simulink model "rmspec"  (Simulink 7.0)
settings: Solver=ode45  StartTime=0.0  StopTime=200  RelTol=1e-3
undefined symbols (not defined in the file): pfb_coeff_gen_calc
libraries: xbsIndex_r4 x3092, casper_library x230, xps_library x24
(part 3 of 33)

== system rmspec/stg3_isel ==
  sync_tvg : Inport
  tvg0 : Inport  Port=2
  tvg1 : Inport  Port=3
  sync_p : Inport  Port=4
  p0 : Inport  Port=5
  p1 : Inport  Port=6
  Constant13 : xbsIndex_r4/Constant  arith_type=Unsigned  const=1  n_bits=32  bin_pt=0  explicit_period=on  period=1  equ=P=C  opselect=C  inp2=PCIN>>17  opr=+  inp1=P  carry=CIN  dbl_ovrd=off  block_type=constant
  Delay1 : xbsIndex_r4/Delay  en=off  latency=1  dbl_ovrd=off  reg_retiming=off  block_type=delay
  Delay24 : xbsIndex_r4/Delay  en=off  latency=1  dbl_ovrd=off  reg_retiming=off  block_type=delay
  Delay3 : xbsIndex_r4/Delay  en=off  latency=1  dbl_ovrd=off  reg_retiming=off  block_type=delay
  Mux : xbsIndex_r4/Mux  inputs=2  en=off  latency=0  precision=Full  arith_type=Unsigned  n_bits=16  bin_pt=14  quantization=Truncate  overflow=Wrap  dbl_ovrd=off  block_type=mux
  Mux1 : xbsIndex_r4/Mux  inputs=2  en=off  latency=0  precision=Full  arith_type=Unsigned  n_bits=16  bin_pt=14  quantization=Truncate  overflow=Wrap  dbl_ovrd=off  block_type=mux
  Mux2 : xbsIndex_r4/Mux  inputs=2  en=off  latency=0  precision=Full  arith_type=Unsigned  n_bits=16  bin_pt=14  quantization=Truncate  overflow=Wrap  dbl_ovrd=off  block_type=mux
  en : xps_library/software register  Tag=xps:sw_reg  SystemSampleTime=-1  io_dir=From Processor  arith_type=Unsigned  bitwidth=32  bin_pt=0  sample_period=1  gw_name=rmspec_stg3_isel_en_user_data_out
      link override pfb1_tv_tge0_rst_user_data_out: arith_type=Unsigned  n_bits=32  bin_pt=0  period=1
      link override pfb1_tv_tgeA_rst_reg_user_data_out: arith_type=Unsigned  n_bits=32  bin_pt=0  period=1
      link override pfb1_tv_tgeA_rst_user_data_out: arith_type=Unsigned  n_bits=32  bin_pt=0  period=1
      link override rmspec_stg3_isel_en_user_data_out: arith_type=Unsigned  n_bits=32  bin_pt=0  period=1
      link override roach_mspec_stg3_isel_en_user_data_out: arith_type=Unsigned  n_bits=32  bin_pt=0  period=1
      link override stg1_stg1_isel_tvg_en_user_data_out: arith_type=Unsigned  n_bits=32  bin_pt=0  period=1
  lsb : xbsIndex_r4/Slice  nbits=1  boolean_output=on  mode=Lower Bit Location + Width  bit1=0  base1=LSB of Input  bit0=0  base0=LSB of Input  dbl_ovrd=off  block_type=slice
      settings: infoedit="Extracts a given range of bits from each input sample and presents it at the output.  The output type is ordinarily unsigned with binary point at zero, but can be Boolean when the slice is one bit wide.<P><P>Hardware notes: In hardware this block costs nothing."  block_version=10.1.3
  sync_o : Outport
  o1 : Outport  Port=2
  o2 : Outport  Port=3
  wires:
  Delay24/1 -> sync_o/1
  [sel] -> Mux/1
  Mux/1 -> Delay24/1
  Delay1/1 -> o1/1
  [sel] -> Mux1/1
  Mux1/1 -> Delay1/1
  Delay3/1 -> o2/1
  [sel] -> Mux2/1
  Mux2/1 -> Delay3/1
  en/1 -> lsb/1
  Constant13/1 -> en/1
  lsb/1 -> [sel]
  p1/1 -> Mux2/2
  tvg1/1 -> Mux2/3
  p0/1 -> Mux1/2
  tvg0/1 -> Mux1/3
  sync_p/1 -> Mux/2
  sync_tvg/1 -> Mux/3

== system rmspec/sys ==
  Constant1 : xbsIndex_r4/Constant  arith_type=Unsigned  const=2^5-1  n_bits=5  bin_pt=0  explicit_period=on  period=1  equ=P=C  opselect=C  inp2=PCIN>>17  opr=+  inp1=P  carry=CIN  dbl_ovrd=off  block_type=constant
  Constant4 : Constant  Value=0  OutDataType=sfix(16)  OutScaling=2^0
  Constant5 : xbsIndex_r4/Constant  arith_type=Unsigned  const=2^5-2  n_bits=5  bin_pt=0  explicit_period=on  period=1  equ=P=C  opselect=C  inp2=PCIN>>17  opr=+  inp1=P  carry=CIN  dbl_ovrd=off  block_type=constant
  Delay18 : xbsIndex_r4/Delay  en=off  latency=1  dbl_ovrd=off  reg_retiming=off  block_type=delay
  Delay19 : xbsIndex_r4/Delay  en=off  latency=1  dbl_ovrd=off  reg_retiming=off  block_type=delay
  Relational : xbsIndex_r4/Relational  mode=a=b  en=off  latency=0  dbl_ovrd=off  block_type=relational
      settings: block_version=10.1.3
  Relational1 : xbsIndex_r4/Relational  mode=a!=b  en=off  latency=0  dbl_ovrd=off  block_type=relational
      settings: block_version=10.1.3
  Slice : xbsIndex_r4/Slice  nbits=1  boolean_output=on  mode=Lower Bit Location + Width  bit1=0  base1=MSB of Input  bit0=0  base0=LSB of Input  dbl_ovrd=off  block_type=slice
      settings: infoedit="Extracts a given range of bits from each input sample and presents it at the output.  The output type is ordinarily unsigned with binary point at zero, but can be Boolean when the slice is one bit wide.<P><P>Hardware notes: In hardware this block costs nothing."  block_version=10.1.3
  reset_reg : xps_library/software register  Tag=xps:sw_reg  SystemSampleTime=-1  io_dir=From Processor  arith_type=Unsigned  bitwidth=32  bin_pt=0  sample_period=1  gw_name=rmspec_sys_reset_reg_user_data_out
      link override qdr_vacc_dram_buf_tv_Subsystem_reset_reg_user_data_out: arith_type=Unsigned  n_bits=32  bin_pt=0  period=1
      link override qdr_vacc_dram_buf_tv_reset_reg_user_data_out: arith_type=Unsigned  n_bits=32  bin_pt=0  period=1
      link override qdr_vacc_dram_buf_tv_sys_reset_reg_user_data_out: arith_type=Unsigned  n_bits=32  bin_pt=0  period=1
      link override qdr_vacc_dram_buf_tv_tvg2_chan_user_data_out: arith_type=Unsigned  n_bits=32  bin_pt=0  period=1
      link override rmspec_sys_reset_reg_user_data_out: arith_type=Unsigned  n_bits=32  bin_pt=0  period=1
      link override roach_mspec_sys_reset_reg_user_data_out: arith_type=Unsigned  n_bits=32  bin_pt=0  period=1
      link override stg1_sys_reset_reg_user_data_out: arith_type=Unsigned  n_bits=32  bin_pt=0  period=1
      link override stg3_backup_sys_reset_reg_user_data_out: arith_type=Unsigned  n_bits=32  bin_pt=0  period=1
      link override stg3_sys_reset_reg_user_data_out: arith_type=Unsigned  n_bits=32  bin_pt=0  period=1
  sync_counter : xbsIndex_r4/Counter  cnt_type=Free Running  cnt_to=15  operation=Up  start_count=0  cnt_by_val=1  arith_type=Unsigned  n_bits=5  bin_pt=0  load_pin=off  rst=on  en=on  explicit_period=on  period=1  dbl_ovrd=off  use_behavioral_HDL=off  use_rpm=off  implementation=Fabric  block_type=counter
  sync : Outport
  rst : Outport  Port=2
  wires:
  sync_counter/1 -> Relational/1, Relational1/1
  Constant5/1 -> Relational/2
  Constant4/1 -> reset_reg/1
  reset_reg/1 -> Slice/1
  Relational/1 -> Delay19/1
  Slice/1 -> sync_counter/1, Delay18/1
  Constant1/1 -> Relational1/2
  Relational1/1 -> sync_counter/2
  Delay18/1 -> rst/1
  Delay19/1 -> sync/1

== system rmspec/tgeC_en ==
  vldi : Inport
  rst : Inport  Port=2
  last : Inport  Port=3
  Constant : xbsIndex_r4/Constant  arith_type=Boolean  const=1  n_bits=1  bin_pt=0  explicit_period=off  period=1  equ=P=C  opselect=C  inp2=PCIN>>17  opr=+  inp1=P  carry=CIN  dbl_ovrd=off  block_type=constant
  Logical : xbsIndex_r4/Logical  logical_function=AND  inputs=2  en=off  latency=0  precision=Full  arith_type=Unsigned  n_bits=16  bin_pt=0  align_bp=on  dbl_ovrd=off  block_type=logical
  Register : xbsIndex_r4/Register  init=0  rst=on  en=on  dbl_ovrd=off  block_type=register
  vldo : Outport
  wires:
  vldi/1 -> Logical/1
  Logical/1 -> vldo/1
  Constant/1 -> Register/1
  rst/1 -> Register/2
  last/1 -> Register/3
  Register/1 -> Logical/2

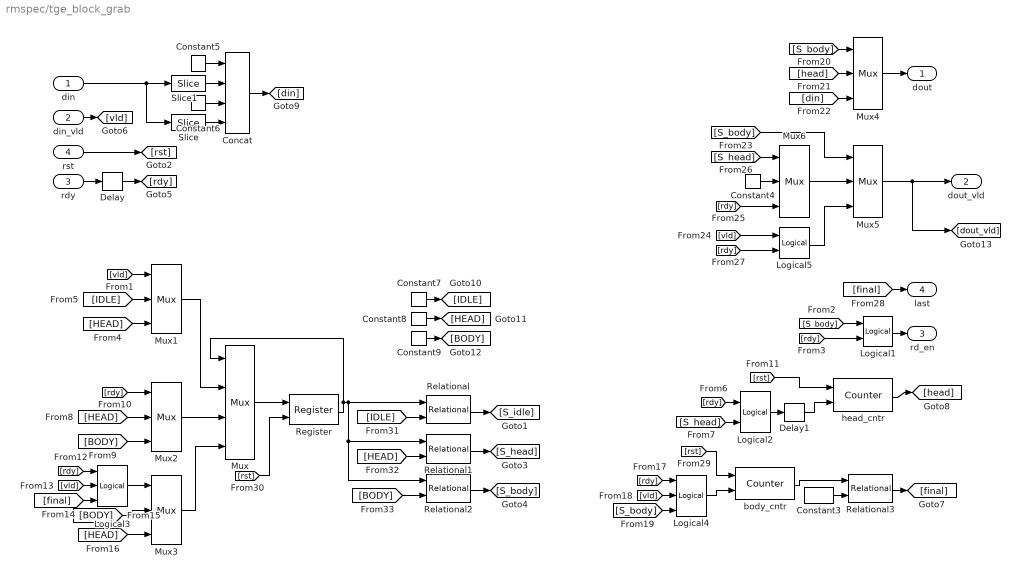
== system rmspec/tge_block_grab ==
  din : Inport
  din_vld : Inport  Port=2
  rdy : Inport  Port=3
  rst : Inport  Port=4
  Concat : xbsIndex_r4/Concat  num_inputs=4  dbl_ovrd=off  block_type=concat
      settings: block_version=10.1.3
  Constant3 : xbsIndex_r4/Constant  arith_type=Unsigned  const=2^9-1  n_bits=9  bin_pt=0  explicit_period=off  period=1  equ=P=C  opselect=C  inp2=PCIN>>17  opr=+  inp1=P  carry=CIN  dbl_ovrd=off  block_type=constant
  Constant4 : xbsIndex_r4/Constant  arith_type=Boolean  const=0  n_bits=2  bin_pt=0  explicit_period=off  period=1  equ=P=C  opselect=C  inp2=PCIN>>17  opr=+  inp1=P  carry=CIN  dbl_ovrd=off  block_type=constant
  Constant5 : xbsIndex_r4/Constant  arith_type=Unsigned  const=0  n_bits=14  bin_pt=0  explicit_period=off  period=1  equ=P=C  opselect=C  inp2=PCIN>>17  opr=+  inp1=P  carry=CIN  dbl_ovrd=off  block_type=constant
  Constant6 : xbsIndex_r4/Constant  arith_type=Unsigned  const=0  n_bits=14  bin_pt=0  explicit_period=off  period=1  equ=P=C  opselect=C  inp2=PCIN>>17  opr=+  inp1=P  carry=CIN  dbl_ovrd=off  block_type=constant
  Constant7 : xbsIndex_r4/Constant  arith_type=Unsigned  const=0  n_bits=2  bin_pt=0  explicit_period=off  period=1  equ=P=C  opselect=C  inp2=PCIN>>17  opr=+  inp1=P  carry=CIN  dbl_ovrd=off  block_type=constant
  Constant8 : xbsIndex_r4/Constant  arith_type=Unsigned  const=1  n_bits=2  bin_pt=0  explicit_period=off  period=1  equ=P=C  opselect=C  inp2=PCIN>>17  opr=+  inp1=P  carry=CIN  dbl_ovrd=off  block_type=constant
  Constant9 : xbsIndex_r4/Constant  arith_type=Unsigned  const=2  n_bits=2  bin_pt=0  explicit_period=off  period=1  equ=P=C  opselect=C  inp2=PCIN>>17  opr=+  inp1=P  carry=CIN  dbl_ovrd=off  block_type=constant
  Delay : xbsIndex_r4/Delay  en=off  latency=1  dbl_ovrd=off  reg_retiming=off  block_type=delay
  Delay1 : xbsIndex_r4/Delay  en=off  latency=1  dbl_ovrd=off  reg_retiming=off  block_type=delay
  Logical1 : xbsIndex_r4/Logical  logical_function=AND  inputs=2  en=off  latency=0  precision=Full  arith_type=Unsigned  n_bits=16  bin_pt=0  align_bp=on  dbl_ovrd=off  block_type=logical
  Logical2 : xbsIndex_r4/Logical  logical_function=AND  inputs=2  en=off  latency=0  precision=Full  arith_type=Unsigned  n_bits=16  bin_pt=0  align_bp=on  dbl_ovrd=off  block_type=logical
  Logical3 : xbsIndex_r4/Logical  logical_function=AND  inputs=3  en=off  latency=0  precision=Full  arith_type=Unsigned  n_bits=16  bin_pt=0  align_bp=on  dbl_ovrd=off  block_type=logical
  Logical4 : xbsIndex_r4/Logical  logical_function=AND  inputs=3  en=off  latency=0  precision=Full  arith_type=Unsigned  n_bits=16  bin_pt=0  align_bp=on  dbl_ovrd=off  block_type=logical
  Logical5 : xbsIndex_r4/Logical  logical_function=AND  inputs=2  en=off  latency=0  precision=Full  arith_type=Unsigned  n_bits=16  bin_pt=0  align_bp=on  dbl_ovrd=off  block_type=logical
  Mux : xbsIndex_r4/Mux  inputs=3  en=off  latency=0  precision=Full  arith_type=Unsigned  n_bits=16  bin_pt=14  quantization=Truncate  overflow=Wrap  dbl_ovrd=off  block_type=mux
  Mux{1..6} (6 alike) : xbsIndex_r4/Mux  inputs=2  en=off  latency=0  precision=Full  arith_type=Unsigned  n_bits=16  bin_pt=14  quantization=Truncate  overflow=Wrap  dbl_ovrd=off  block_type=mux
  Register : xbsIndex_r4/Register  init=0  rst=on  en=off  dbl_ovrd=off  block_type=register
  Relational{,1..3} (4 alike) : xbsIndex_r4/Relational  mode=a=b  en=off  latency=0  dbl_ovrd=off  block_type=relational
      settings: block_version=10.1.3
  Slice : xbsIndex_r4/Slice  nbits=18  boolean_output=off  mode=Lower Bit Location + Width  bit1=0  base1=LSB of Input  bit0=0  base0=LSB of Input  dbl_ovrd=off  block_type=slice
      settings: infoedit="Extracts a given range of bits from each input sample and presents it at the output.  The output type is ordinarily unsigned with binary point at zero, but can be Boolean when the slice is one bit wide.<P><P>Hardware notes: In hardware this block costs nothing."  block_version=10.1.3
  Slice1 : xbsIndex_r4/Slice  nbits=18  boolean_output=off  mode=Lower Bit Location + Width  bit1=0  base1=LSB of Input  bit0=18  base0=LSB of Input  dbl_ovrd=off  block_type=slice
      settings: infoedit="Extracts a given range of bits from each input sample and presents it at the output.  The output type is ordinarily unsigned with binary point at zero, but can be Boolean when the slice is one bit wide.<P><P>Hardware notes: In hardware this block costs nothing."  block_version=10.1.3
  body_cntr : xbsIndex_r4/Counter  cnt_type=Free Running  cnt_to=Inf  operation=Up  start_count=0  cnt_by_val=1  arith_type=Unsigned  n_bits=9  bin_pt=0  load_pin=off  rst=on  en=on  explicit_period=on  period=1  dbl_ovrd=off  use_behavioral_HDL=off  use_rpm=off  implementation=Fabric  block_type=counter
  head_cntr : xbsIndex_r4/Counter  cnt_type=Free Running  cnt_to=Inf  operation=Up  start_count=0  cnt_by_val=1  arith_type=Unsigned  n_bits=64  bin_pt=0  load_pin=off  rst=on  en=on  explicit_period=on  period=1  dbl_ovrd=off  use_behavioral_HDL=off  use_rpm=off  implementation=Fabric  block_type=counter
  dout : Outport
  dout_vld : Outport  Port=2
  rd_en : Outport  Port=3
  last : Outport  Port=4
  wires:
  Register/1 -> Relational2/1, Relational1/1, Relational/1, Mux/1
  Relational/1 -> [S_idle]
  Relational1/1 -> [S_head]
  Relational2/1 -> [S_body]
  rdy/1 -> Delay/1
  [rdy] -> Logical1/2
  Logical1/1 -> rd_en/1
  Logical2/1 -> Delay1/1
  Delay/1 -> [rdy]
  [S_body] -> Logical1/1
  [rdy] -> Logical2/1
  [S_head] -> Logical2/2
  Mux/1 -> Register/1
  din_vld/1 -> [vld]
  [vld] -> Mux1/1
  [HEAD] -> Mux1/3
  [IDLE] -> Mux1/2
  Mux1/1 -> Mux/2
  Mux2/1 -> Mux/3
  [HEAD] -> Mux2/2
  [BODY] -> Mux2/3
  [rdy] -> Mux2/1
  [rdy] -> Logical3/1
  [vld] -> Logical3/2
  [final] -> Logical3/3
  Logical3/1 -> Mux3/1
  [BODY] -> Mux3/2
  [HEAD] -> Mux3/3
  head_cntr/1 -> [head]
  Constant3/1 -> Relational3/2
  body_cntr/1 -> Relational3/1
  [rdy] -> Logical4/1
  [vld] -> Logical4/2
  [S_body] -> Logical4/3
  Relational3/1 -> [final]
  Mux3/1 -> Mux/4
  [S_body] -> Mux4/1
  [head] -> Mux4/2
  [din] -> Mux4/3
  Mux4/1 -> dout/1
  [S_body] -> Mux5/1
  Mux5/1 -> dout_vld/1, [dout_vld]
  Mux6/1 -> Mux5/2
  [S_head] -> Mux6/1
  Constant4/1 -> Mux6/2
  [rdy] -> Logical5/2
  [vld] -> Logical5/1
  Logical5/1 -> Mux5/3
  [rdy] -> Mux6/3
  [final] -> last/1
  Concat/1 -> [din]
  Slice1/1 -> Concat/2
  Constant5/1 -> Concat/1
  Constant6/1 -> Concat/3
  din/1 -> Slice1/1, Slice/1
  Slice/1 -> Concat/4
  Constant7/1 -> [IDLE]
  Constant8/1 -> [HEAD]
  Constant9/1 -> [BODY]
  [IDLE] -> Relational/2
  [HEAD] -> Relational1/2
  [BODY] -> Relational2/2
  rst/1 -> [rst]
  [rst] -> head_cntr/1
  Delay1/1 -> head_cntr/2
  [rst] -> body_cntr/1
  Logical4/1 -> body_cntr/2
  [rst] -> Register/2

== system rmspec/tvg1 ==
  AddSub : xbsIndex_r4/AddSub  mode=Addition  use_carryin=off  use_carryout=off  en=off  latency=0  precision=User Defined  arith_type=Unsigned  n_bits=12  bin_pt=0  quantization=Truncate  overflow=Wrap  dbl_ovrd=off  use_behavioral_HDL=on  pipelined=off  use_rpm=on  hw_selection=Fabric  block_type=addsub
      settings: block_version=10.1.3
  Constant : xbsIndex_r4/Constant  arith_type=Unsigned  const=2^27-1  n_bits=28  bin_pt=0  explicit_period=off  period=1  equ=P=C  opselect=C  inp2=PCIN>>17  opr=+  inp1=P  carry=CIN  dbl_ovrd=off  block_type=constant
  ROM0 : xbsIndex_r4/ROM  depth=4096  initVector=lev*sin((pi/2048)*(0:4:4096*4-1))  distributed_mem=Block RAM  rst=off  init_reg=0  en=off  latency=1  arith_type="Signed  (2's comp)"  n_bits=8  bin_pt=7  dbl_ovrd=off  optimize=Area  use_rpm=on  block_type=sprom
      settings: block_version=10.1.3
  ROM1 : xbsIndex_r4/ROM  depth=4096  initVector=lev*sin((pi/2048)*(1:4:4096*4-1))  distributed_mem=Block RAM  rst=off  init_reg=0  en=off  latency=1  arith_type="Signed  (2's comp)"  n_bits=8  bin_pt=7  dbl_ovrd=off  optimize=Area  use_rpm=on  block_type=sprom
      settings: block_version=10.1.3
  ROM2 : xbsIndex_r4/ROM  depth=4096  initVector=lev*sin((pi/2048)*(2:4:4096*4-1))  distributed_mem=Block RAM  rst=off  init_reg=0  en=off  latency=1  arith_type="Signed  (2's comp)"  n_bits=8  bin_pt=7  dbl_ovrd=off  optimize=Area  use_rpm=on  block_type=sprom
      settings: block_version=10.1.3
  ROM3 : xbsIndex_r4/ROM  depth=4096  initVector=lev*sin((pi/2048)*(3:4:4096*4-1))  distributed_mem=Block RAM  rst=off  init_reg=0  en=off  latency=1  arith_type="Signed  (2's comp)"  n_bits=8  bin_pt=7  dbl_ovrd=off  optimize=Area  use_rpm=on  block_type=sprom
      settings: block_version=10.1.3
  Relational : xbsIndex_r4/Relational  mode=a=b  en=off  latency=1  dbl_ovrd=off  block_type=relational
      settings: block_version=10.1.3
  addr : xbsIndex_r4/Register  init=0  rst=off  en=off  dbl_ovrd=off  block_type=register
  tick_counter : xbsIndex_r4/Counter  cnt_type=Free Running  cnt_to=Inf  operation=Up  start_count=0  cnt_by_val=1  arith_type=Unsigned  n_bits=28  bin_pt=0  load_pin=off  rst=off  en=off  explicit_period=on  period=1  dbl_ovrd=off  use_behavioral_HDL=off  use_rpm=off  implementation=Fabric  block_type=counter
  tick_counter1 : xbsIndex_r4/Counter  cnt_type=Free Running  cnt_to=Inf  operation=Up  start_count=128  cnt_by_val=1  arith_type=Unsigned  n_bits=10  bin_pt=0  load_pin=off  rst=off  en=on  explicit_period=on  period=1  dbl_ovrd=off  use_behavioral_HDL=off  use_rpm=off  implementation=Fabric  block_type=counter
  Out1 : Outport
  Out2 : Outport  Port=2
  Out3 : Outport  Port=3
  Out4 : Outport  Port=4
  wires:
  ROM0/1 -> Out1/1
  ROM1/1 -> Out2/1
  ROM2/1 -> Out3/1
  ROM3/1 -> Out4/1
  tick_counter/1 -> Relational/1
  Constant/1 -> Relational/2
  Relational/1 -> tick_counter1/1
  AddSub/1 -> addr/1
  tick_counter1/1 -> AddSub/1
  addr/1 -> AddSub/2, ROM2/1, ROM3/1, ROM1/1, ROM0/1

== system rmspec/tvg2 ==
  sync : Inport  OutDataType=sfix(16)  OutScaling=2^0
  Constant : xbsIndex_r4/Constant  arith_type=Signed (2's comp)  const=0  n_bits=9  bin_pt=8  explicit_period=on  period=1  equ=P=C  opselect=C  inp2=PCIN>>17  opr=+  inp1=P  carry=CIN  dbl_ovrd=off  block_type=constant
  Delay : xbsIndex_r4/Delay  en=off  latency=1  dbl_ovrd=off  reg_retiming=off  block_type=delay
  Delay1 : xbsIndex_r4/Delay  en=off  latency=1  dbl_ovrd=off  reg_retiming=off  block_type=delay
  Delay2 : xbsIndex_r4/Delay  en=off  latency=3  dbl_ovrd=off  reg_retiming=off  block_type=delay
  Delay3 : xbsIndex_r4/Delay  en=off  latency=1  dbl_ovrd=off  reg_retiming=off  block_type=delay
  Delay4 : xbsIndex_r4/Delay  en=off  latency=2  dbl_ovrd=off  reg_retiming=off  block_type=delay
  Mult : xbsIndex_r4/Mult  precision=User Defined  arith_type=Unsigned  n_bits=12  bin_pt=0  quantization=Truncate  overflow=Wrap  en=off  latency=3  dbl_ovrd=off  use_behavioral_HDL=off  use_embedded=on  opt=Speed  optimum_pipeline=off  pipeline=on  use_rpm=on  placement_style=Triangular  block_type=mult
      settings: infoedit=Hardware notes: To use the internal pipeline stage of the dedicated multiplier you must select 'Pipeline for maximum performance'.  block_version=10.1.3
  Shift : xbsIndex_r4/Shift  shift_dir=Right  shift_bits=6  en=off  latency=1  precision=User Defined  arith_type="Signed  (2's comp)"  n_bits=9  bin_pt=8  quantization="Round  (unbiased: +/- Inf)"  overflow=Wrap  dbl_ovrd=off  block_type=shift
      settings: block_version=10.1.3
  chan_s : xbsIndex_r4/Slice  nbits=9  boolean_output=off  mode=Lower Bit Location + Width  bit1=0  base1=LSB of Input  bit0=10  base0=LSB of Input  dbl_ovrd=off  block_type=slice
      settings: infoedit="Extracts a given range of bits from each input sample and presents it at the output.  The output type is ordinarily unsigned with binary point at zero, but can be Boolean when the slice is one bit wide.<P><P>Hardware notes: In hardware this block costs nothing."  block_version=10.1.3
  chan_s1 : xbsIndex_r4/Slice  nbits=10  boolean_output=off  mode=Lower Bit Location + Width  bit1=0  base1=LSB of Input  bit0=0  base0=LSB of Input  dbl_ovrd=off  block_type=slice
      settings: infoedit="Extracts a given range of bits from each input sample and presents it at the output.  The output type is ordinarily unsigned with binary point at zero, but can be Boolean when the slice is one bit wide.<P><P>Hardware notes: In hardware this block costs nothing."  block_version=10.1.3
  progress : xbsIndex_r4/Counter  cnt_type=Free Running  cnt_to=Inf  operation=Up  start_count=0  cnt_by_val=1  arith_type=Unsigned  n_bits=19  bin_pt=0  load_pin=off  rst=on  en=off  explicit_period=on  period=1  dbl_ovrd=off  use_behavioral_HDL=off  use_rpm=off  implementation=Fabric  block_type=counter
  ri_to_c : casper_library/Misc/ri_to_c  SystemSampleTime=-1
  ri_to_c1 : casper_library/Misc/ri_to_c  SystemSampleTime=-1
  tvg_lookup : xbsIndex_r4/ROM  depth=4096  initVector=cos(pi*(0:4065)/128)  distributed_mem=Block RAM  rst=off  init_reg=0  en=off  latency=2  arith_type="Signed  (2's comp)"  n_bits=9  bin_pt=8  dbl_ovrd=off  optimize=Area  use_rpm=on  block_type=sprom
      settings: block_version=10.1.3
  sync_o : Outport
  Out1 : Outport  Port=2
  Out2 : Outport  Port=3
  wires:
  progress/1 -> chan_s/1, chan_s1/1
  chan_s/1 -> [chan]
  chan_s1/1 -> [samp]
  ri_to_c/1 -> Out1/1
  ri_to_c1/1 -> Out2/1
  Constant/1 -> ri_to_c/2, ri_to_c1/1
  tvg_lookup/1 -> Shift/1
  Delay/1 -> ri_to_c/1, ri_to_c1/2
  sync/1 -> progress/1, Delay2/1
  Delay3/1 -> Delay1/1
  Delay1/1 -> sync_o/1
  [chan] -> Mult/1
  [samp] -> Mult/2
  Mult/1 -> tvg_lookup/1
  Delay2/1 -> Delay4/1
  Shift/1 -> Delay/1
  Delay4/1 -> Delay3/1

== system rmspec/tvg3 ==
  sync : Inport  OutDataType=sfix(16)  OutScaling=2^0
  AddSub1 : xbsIndex_r4/AddSub  mode=Subtraction  use_carryin=off  use_carryout=off  en=off  latency=2  precision=Full  arith_type=Unsigned  n_bits=16  bin_pt=14  quantization=Truncate  overflow=Wrap  dbl_ovrd=off  use_behavioral_HDL=off  pipelined=off  use_rpm=on  hw_selection=Fabric  block_type=addsub
      settings: block_version=10.1.3
  Constant : Constant  Value=3200  OutDataType=sfix(16)  OutScaling=2^0
  Constant1 : xbsIndex_r4/Constant  arith_type=Unsigned  const=128  n_bits=7  bin_pt=0  explicit_period=on  period=1  equ=P=C  opselect=C  inp2=PCIN>>17  opr=+  inp1=P  carry=CIN  dbl_ovrd=off  block_type=constant
  Constant2 : xbsIndex_r4/Constant  arith_type=Unsigned  const=128  n_bits=7  bin_pt=0  explicit_period=on  period=1  equ=P=C  opselect=C  inp2=PCIN>>17  opr=+  inp1=P  carry=CIN  dbl_ovrd=off  block_type=constant
  Constant3 : xbsIndex_r4/Constant  arith_type=Unsigned  const=63  n_bits=6  bin_pt=0  explicit_period=on  period=1  equ=P=C  opselect=C  inp2=PCIN>>17  opr=+  inp1=P  carry=CIN  dbl_ovrd=off  block_type=constant
  Convert : xbsIndex_r4/Convert  arith_type=Unsigned  n_bits=vaccwidth  bin_pt=0  quantization=Truncate  overflow=Wrap  latency=0  dbl_ovrd=off  pipeline=off  block_type=convert
      settings: block_version=10.1.3
  Convert1 : xbsIndex_r4/Convert  arith_type=Unsigned  n_bits=vaccwidth  bin_pt=0  quantization=Truncate  overflow=Wrap  latency=0  dbl_ovrd=off  pipeline=off  block_type=convert
      settings: block_version=10.1.3
  Delay1 : xbsIndex_r4/Delay  en=off  latency=1  dbl_ovrd=off  reg_retiming=off  block_type=delay
  Delay2 : xbsIndex_r4/Delay  en=off  latency=1  dbl_ovrd=off  reg_retiming=off  block_type=delay
  Delay3 : xbsIndex_r4/Delay  en=off  latency=1  dbl_ovrd=off  reg_retiming=off  block_type=delay
  Delay4 : xbsIndex_r4/Delay  en=off  latency=2  dbl_ovrd=off  reg_retiming=off  block_type=delay
  Delay5 : xbsIndex_r4/Delay  en=off  latency=2  dbl_ovrd=off  reg_retiming=off  block_type=delay
  Inverter : xbsIndex_r4/Inverter  en=off  latency=0  dbl_ovrd=off  block_type=inv
  Logical : xbsIndex_r4/Logical  logical_function=AND  inputs=2  en=off  latency=1  precision=Full  arith_type=Unsigned  n_bits=16  bin_pt=0  align_bp=on  dbl_ovrd=off  block_type=logical
  Logical1 : xbsIndex_r4/Logical  logical_function=AND  inputs=2  en=off  latency=1  precision=Full  arith_type=Unsigned  n_bits=16  bin_pt=0  align_bp=on  dbl_ovrd=off  block_type=logical
  Logical2 : xbsIndex_r4/Logical  logical_function=AND  inputs=2  en=off  latency=0  precision=Full  arith_type=Unsigned  n_bits=16  bin_pt=0  align_bp=on  dbl_ovrd=off  block_type=logical
  Mux : xbsIndex_r4/Mux  inputs=2  en=off  latency=0  precision=Full  arith_type=Unsigned  n_bits=16  bin_pt=14  quantization=Truncate  overflow=Wrap  dbl_ovrd=off  block_type=mux
  Mux1 : xbsIndex_r4/Mux  inputs=2  en=off  latency=0  precision=Full  arith_type=Unsigned  n_bits=16  bin_pt=14  quantization=Truncate  overflow=Wrap  dbl_ovrd=off  block_type=mux
  Relational : xbsIndex_r4/Relational  mode=a=b  en=off  latency=1  dbl_ovrd=off  block_type=relational
      settings: block_version=10.1.3
  Relational1 : xbsIndex_r4/Relational  mode=a=b  en=off  latency=1  dbl_ovrd=off  block_type=relational
      settings: block_version=10.1.3
  Slice1 : xbsIndex_r4/Slice  nbits=fftsize-4  boolean_output=off  mode=Lower Bit Location + Width  bit1=0  base1=LSB of Input  bit0=4  base0=LSB of Input  dbl_ovrd=off  block_type=slice
      settings: infoedit="Extracts a given range of bits from each input sample and presents it at the output.  The output type is ordinarily unsigned with binary point at zero, but can be Boolean when the slice is one bit wide.<P><P>Hardware notes: In hardware this block costs nothing."  block_version=10.1.3
  Slice2 : xbsIndex_r4/Slice  nbits=1  boolean_output=on  mode=Lower Bit Location + Width  bit1=0  base1=LSB of Input  bit0=10  base0=LSB of Input  dbl_ovrd=off  block_type=slice
      settings: infoedit="Extracts a given range of bits from each input sample and presents it at the output.  The output type is ordinarily unsigned with binary point at zero, but can be Boolean when the slice is one bit wide.<P><P>Hardware notes: In hardware this block costs nothing."  block_version=10.1.3
  Slice3 : xbsIndex_r4/Slice  nbits=10-1  boolean_output=off  mode=Lower Bit Location + Width  bit1=0  base1=LSB of Input  bit0=11  base0=LSB of Input  dbl_ovrd=off  block_type=slice
      settings: infoedit="Extracts a given range of bits from each input sample and presents it at the output.  The output type is ordinarily unsigned with binary point at zero, but can be Boolean when the slice is one bit wide.<P><P>Hardware notes: In hardware this block costs nothing."  block_version=10.1.3
  Slice4 : xbsIndex_r4/Slice  nbits=fftsize  boolean_output=off  mode=Lower Bit Location + Width  bit1=0  base1=LSB of Input  bit0=0  base0=LSB of Input  dbl_ovrd=off  block_type=slice
      settings: infoedit="Extracts a given range of bits from each input sample and presents it at the output.  The output type is ordinarily unsigned with binary point at zero, but can be Boolean when the slice is one bit wide.<P><P>Hardware notes: In hardware this block costs nothing."  block_version=10.1.3
  Slice5 : xbsIndex_r4/Slice  nbits=fftsize  boolean_output=off  mode=Lower Bit Location + Width  bit1=0  base1=LSB of Input  bit0=0  base0=LSB of Input  dbl_ovrd=off  block_type=slice
      settings: infoedit="Extracts a given range of bits from each input sample and presents it at the output.  The output type is ordinarily unsigned with binary point at zero, but can be Boolean when the slice is one bit wide.<P><P>Hardware notes: In hardware this block costs nothing."  block_version=10.1.3
  Slice6 : xbsIndex_r4/Slice  nbits=nochan-1  boolean_output=off  mode=Lower Bit Location + Width  bit1=0  base1=LSB of Input  bit0=fftsize  base0=LSB of Input  dbl_ovrd=off  block_type=slice
      settings: infoedit="Extracts a given range of bits from each input sample and presents it at the output.  The output type is ordinarily unsigned with binary point at zero, but can be Boolean when the slice is one bit wide.<P><P>Hardware notes: In hardware this block costs nothing."  block_version=10.1.3
  progress : xbsIndex_r4/Counter  cnt_type=Free Running  cnt_to=Inf  operation=Up  start_count=0  cnt_by_val=1  arith_type=Unsigned  n_bits=fftsize + nochan - 1  bin_pt=0  load_pin=off  rst=on  en=off  explicit_period=on  period=1  dbl_ovrd=off  use_behavioral_HDL=off  use_rpm=off  implementation=Fabric  block_type=counter
  tvg2_chan : xps_library/software register  Tag=xps:sw_reg  SystemSampleTime=-1  io_dir=From Processor  arith_type=Unsigned  bitwidth=32  bin_pt=0  sample_period=1  gw_name=rmspec_tvg3_tvg2_chan_user_data_out
      link override qdr_vacc_dram_buf_tv_tvg2_chan_user_data_out: arith_type=Unsigned  n_bits=32  bin_pt=0  period=1
      link override rmspec_tvg3_tvg2_chan_user_data_out: arith_type=Unsigned  n_bits=32  bin_pt=0  period=1
      link override roach_mspec_tvg3_tvg2_chan_user_data_out: arith_type=Unsigned  n_bits=32  bin_pt=0  period=1
      link override stg3_backup_tvg2_chan_user_data_out: arith_type=Unsigned  n_bits=32  bin_pt=0  period=1
      link override stg3_tvg2_chan_user_data_out: arith_type=Unsigned  n_bits=32  bin_pt=0  period=1
  sync_o : Outport
  Out1 : Outport  Port=2
  Out2 : Outport  Port=3
  wires:
  sync/1 -> progress/1, Delay4/1
  Delay3/1 -> sync_o/1
  Delay1/1 -> Out1/1
  progress/1 -> Slice1/1, Slice5/1, Slice6/1
  Slice1/1 -> Delay5/1, AddSub1/2
  Delay4/1 -> Delay3/1
  Constant3/1 -> AddSub1/1
  Delay2/1 -> Out2/1
  Convert1/1 -> Delay1/1
  Convert/1 -> Delay2/1
  tvg2_chan/1 -> Slice2/1, Slice3/1, Slice4/1
  Mux/1 -> Convert/1
  Constant1/1 -> Mux/3
  Logical1/1 -> Mux1/1
  Logical/1 -> Mux/1
  Delay5/1 -> Mux1/2
  Constant2/1 -> Mux1/3
  AddSub1/1 -> Mux/2
  Slice2/1 -> Logical/2, Inverter/1
  Inverter/1 -> Logical1/2
  Slice5/1 -> Relational/1
  Slice4/1 -> Relational/2
  Slice6/1 -> Relational1/1
  Slice3/1 -> Relational1/2
  Relational/1 -> Logical2/1
  Relational1/1 -> Logical2/2
  Logical2/1 -> Logical1/1, Logical/1
  Mux1/1 -> Convert1/1
  Constant/1 -> tvg2_chan/1

== system rmspec/w_fft ==
  sync : Inport
  i0 : Inport  Port=2
  i1 : Inport  Port=3
  " window" : Subsystem  mask{wintype=0, size=10, coeff_width=18, o_width=25, i_width=9}
      mask prompts: wintype "Windowing Function:"; size "size (2^n)"; coeff_width "coeff width"; o_width "out width"; i_width "in width"
  Constant4 : xbsIndex_r4/Constant  arith_type=Unsigned  const=1023  n_bits=10  bin_pt=0  explicit_period=on  period=1  equ=P=C  opselect=C  inp2=PCIN>>17  opr=+  inp1=P  carry=CIN  dbl_ovrd=off  block_type=constant
  Delay{,1..3} (4 alike) : xbsIndex_r4/Delay  en=off  latency=1  dbl_ovrd=off  reg_retiming=off  block_type=delay
  Shift{1..4} (4 alike) : xbsIndex_r4/Shift  shift_dir=Right  shift_bits=1  en=off  latency=1  precision=Full  arith_type="Signed  (2's comp)"  n_bits=16  bin_pt=14  quantization=Truncate  overflow=Wrap  dbl_ovrd=off  block_type=shift
      settings: block_version=10.1.3
  c_to_ri : casper_library/Misc/c_to_ri  SystemSampleTime=-1  n_bits=25  bin_pt=24
      settings: AttributesFormatString=25_24 r/i
  c_to_ri1 : casper_library/Misc/c_to_ri  SystemSampleTime=-1  n_bits=25  bin_pt=24
      settings: AttributesFormatString=25_24 r/i
  fft : Subsystem  AncestorBlock=casper_library/FFTs/fft  mask(fft){FFTSize=10, input_bit_width=25, coeff_bit_width=18, n_inputs=0, quantization=Truncate, overflow=Wrap, add_latency=3, mult_latency=3, bram_latency=2, arch=Virtex5, opt_target=Logic, coeffs_bit_limit=8, delays_bit_limit=9, specify_mult=off, mult_spec=[0 1 1 2 1 1 1 1 1 1]}
      mask prompts: FFTSize "Size of FFT: (2^?)"; input_bit_width "Input/Output Bit Width"; coeff_bit_width "Coefficient Bit Width"; n_inputs "Number of Simultaneous Inputs: (2^?)"; quantization "Quantization Behavior"; overflow "Overflow Behavior"; add_latency "Add Latency"; mult_latency "Mult Latency"; bram_latency "BRAM Latency"; arch "Architecture"; opt_target "Optimisation Target"; coeffs_bit_limit "Number bits above which to store stage's coefficients in BRAM (2^? bits)"; delays_bit_limit "Number bits above which to store stage's delays in BRAM (2^? bits)"; specify_mult "Specify multiplier use (behavioral HDL if not specified)"; mult_spec "Multiplier specification (0=core, 1=embedded, 2=behavioural) (left=1st stage)"
      mask init:
      | fft_init(gcb,...
      |     'FFTSize', FFTSize, ...
      |     'input_bit_width', input_bit_width, ...
      |     'coeff_bit_width', coeff_bit_width, ...
      |     'n_inputs', n_inputs, ...
      |     'quantization', quantization, ...
      |     'overflow', overflow, ...
      |     'add_latency', add_latency, ...
      |     'mult_latency', mult_latency, ...
      |     'bram_latency', bram_latency, ...
      |     'arch', arch, ...
      |     'opt_target', opt_target, ...
      |     'coeffs_bit_limit', coeffs_bit_limit, ...
      |     'delays_bit_limit', delays_bit_limit, ...
      |     'specify_mult', specify_mult, ...
      |     'mult_spec', mult_spec);
      settings: AttributesFormatString=FFTSize=10, n_inputs=0
      mask Help: eval('xlWeb([getenv(''MLIB_ROOT''), ''\doc\htmlblocks\sp_fft\sp_fft.html''])')
      mask StyleString: edit,edit,edit,edit,popup(Truncate|Round  (unbiased: +/- Inf)|Round  (unbiased: Even Values)),popup(Wrap|Saturate|Error),edit,edit,edit,popup(Virtex2Pro|Virtex5),popup(Logic|Multipliers),edit,edit,checkbox,edit
      mask CallbackString:
      | % fft_size = eval(get_param(gcb, 'FFTSize'));
      | % old_vec = eval(get_param(gcb, 'mult_spec'));
      | 
      | % vec = 2.*ones(1,fft_size);
      | % old_size = length(old_vec);
      | 
      | % if(old_size <= fft_size), size = old_size;
      | % else, size = fft_size;
      | % end
      | 
      | % for n = 1:size, vec(n) = old_vec(n); end
      | % set_param(gcb, 'mult_spec', mat2str(vec));|||||||||||||specify_mult = get_param(gcb,'specify_mult');
      | visibs = get_param(gcb, 'MaskVisibilities');
      | if( strcmp(specify_mult,'off')), visibs{15} = 'off';
      | else visibs{15} = 'on';
      | end
      | set_param(gcb, 'MaskVisibilities', visibs);
      | 
      | |% vec = eval( get_param(gcb, 'mult_spec'));
      | % vec_size = length(vec);
      | % fft_size = eval( get_param(gcb, 'FFTSize'));
      | % new_vec = 2.*ones(1, fft_size);
      | 
      | % if(vec_size <= fft_size), size = vec_size;
      | % else size = fft_size;
      | % end
      | 
      | % for n=1:size,
      | %    new_vec(n) = vec(n);
      | % end
      | % set_param(gcb, 'mult_spec', mat2str(new_vec));
  ri_to_c : casper_library/Misc/ri_to_c  SystemSampleTime=-1
  ri_to_c1 : casper_library/Misc/ri_to_c  SystemSampleTime=-1
  sync_o : Outport
  o0 : Outport  Port=2
  o1 : Outport  Port=3
  of : Outport  Port=4
  wires:
  " window"/3(pol1_o) -> c_to_ri1/1
  " window"/2(pol0_o) -> c_to_ri/1
  " window"/1(sync_o) -> Delay/1
  ri_to_c1/1 -> Delay3/1
  Shift2/1 -> ri_to_c1/2
  Shift4/1 -> ri_to_c1/1
  c_to_ri1/2 -> Shift2/1
  c_to_ri1/1 -> Shift4/1
  ri_to_c/1 -> Delay2/1
  Shift1/1 -> ri_to_c/2
  Shift3/1 -> ri_to_c/1
  c_to_ri/2 -> Shift1/1
  c_to_ri/1 -> Shift3/1
  Delay/1 -> Delay1/1
  sync/1 -> " window"/1(sync)
  fft/3(out1) -> o1/1
  fft/2(out0) -> o0/1
  fft/1(sync_out) -> sync_o/1
  Constant4/1 -> fft/2(shift)
  i1/1 -> " window"/3(pol1_i)
  i0/1 -> " window"/2(pol0_i)
  Delay1/1 -> fft/1(sync)
  Delay2/1 -> fft/3(pol0)
  Delay3/1 -> fft/4(pol1)
  fft/4(of) -> of/1

== system rmspec/bram_vacc/simple_bram_vacc ==
  new_acc : Inport  OutDataType=sfix(16)  OutScaling=2^0
  din : Inport  Port=2  OutDataType=sfix(16)  OutScaling=2^0
  Adder0 : xbsIndex_r4/AddSub  mode=Addition  use_carryin=off  use_carryout=off  en=off  latency=2  precision=User Defined  arith_type="Signed  (2's comp)"  n_bits=n_bits  bin_pt=bin_pos  quantization=Truncate  overflow=Wrap  dbl_ovrd=off  use_behavioral_HDL=on  pipelined=off  use_rpm=on  hw_selection=Fabric  block_type=addsub
      settings: xl_area=[0, 0, 0, 0, 0, 0, 0]  block_version=10.1.3
  Delay1 : xbsIndex_r4/Delay  en=off  latency=1  dbl_ovrd=off  reg_retiming=off  block_type=delay
  Delay2 : xbsIndex_r4/Delay  en=off  latency=1  dbl_ovrd=off  reg_retiming=off  block_type=delay
  Mux0 : xbsIndex_r4/Mux  inputs=2  en=off  latency=0  precision=Full  arith_type="Signed  (2's comp)"  n_bits=8  bin_pt=2  quantization=Truncate  overflow=Wrap  dbl_ovrd=off  block_type=mux
      settings: xl_area=[0, 0, 0, 0, 0, 0, 0]
  delay_bram : Subsystem  mask(delay_bram){DelayLen=n_chans - 2 - 1, bram_latency=2}
      mask prompts: DelayLen "Delay By:"; bram_latency "BRAM Latency"
      mask help: A delay block that uses BRAM for its storage.
      mask init:
      | if (DelayLen <= bram_latency)
      | 	error('delay value must be greater than BRAM Latency');
      | end
      | BitWidth = max(ceil(log2(DelayLen)), 2);
      mask Help: eval('xlWeb([getenv(''MLIB_ROOT''), ''\doc\html\sp_delay_bram\sp_delay_bram.html''])')
  pulse_ext : Subsystem  mask(pulse_ext){pulse_len=n_chans}
      mask prompts: pulse_len "Length of Pulse"
      mask help:
      | Extends a boolean signal to be high for the specified number of clocks after
      | the last high input.
      mask init:
      | bits = ceil(log2(pulse_len+1));
      mask Help: eval('xlWeb([getenv(''MLIB_ROOT''), ''\casper_library\doc\pulse_ext_usage.html''])')
  zero : xbsIndex_r4/Constant  arith_type=Signed (2's comp)  const=0  n_bits=32  bin_pt=6  explicit_period=on  period=1  equ=P=C  opselect=C  inp2=PCIN>>17  opr=+  inp1=P  carry=CIN  dbl_ovrd=off  block_type=constant
  dout : Outport  OutDataType=sfix(16)  OutScaling=2^0
  valid : Outport  Port=2  OutDataType=sfix(16)  OutScaling=2^0
  wires:
  zero/1 -> Mux0/3
  Mux0/1 -> Delay2/1
  pulse_ext/1(out) -> Mux0/1, valid/1
  din/1 -> Delay1/1
  new_acc/1 -> pulse_ext/1(in)
  delay_bram/1(Out1) -> Mux0/2, dout/1
  Adder0/1 -> delay_bram/1(In1)
  Delay1/1 -> Adder0/1
  Delay2/1 -> Adder0/2

== system rmspec/bram_vacc/simple_bram_vacc1 ==
  new_acc : Inport  OutDataType=sfix(16)  OutScaling=2^0
  din : Inport  Port=2  OutDataType=sfix(16)  OutScaling=2^0
  Adder0 : xbsIndex_r4/AddSub  mode=Addition  use_carryin=off  use_carryout=off  en=off  latency=2  precision=User Defined  arith_type="Signed  (2's comp)"  n_bits=n_bits  bin_pt=bin_pos  quantization=Truncate  overflow=Wrap  dbl_ovrd=off  use_behavioral_HDL=on  pipelined=off  use_rpm=on  hw_selection=Fabric  block_type=addsub
      settings: xl_area=[0, 0, 0, 0, 0, 0, 0]  block_version=10.1.3
  Delay1 : xbsIndex_r4/Delay  en=off  latency=1  dbl_ovrd=off  reg_retiming=off  block_type=delay
  Delay2 : xbsIndex_r4/Delay  en=off  latency=1  dbl_ovrd=off  reg_retiming=off  block_type=delay
  Mux0 : xbsIndex_r4/Mux  inputs=2  en=off  latency=0  precision=Full  arith_type="Signed  (2's comp)"  n_bits=8  bin_pt=2  quantization=Truncate  overflow=Wrap  dbl_ovrd=off  block_type=mux
      settings: xl_area=[0, 0, 0, 0, 0, 0, 0]
  delay_bram : Subsystem  mask(delay_bram){DelayLen=n_chans - 2 - 1, bram_latency=2}
      mask prompts: DelayLen "Delay By:"; bram_latency "BRAM Latency"
      mask help: A delay block that uses BRAM for its storage.
      mask init:
      | if (DelayLen <= bram_latency)
      | 	error('delay value must be greater than BRAM Latency');
      | end
      | BitWidth = max(ceil(log2(DelayLen)), 2);
      mask Help: eval('xlWeb([getenv(''MLIB_ROOT''), ''\doc\html\sp_delay_bram\sp_delay_bram.html''])')
  pulse_ext : Subsystem  mask(pulse_ext){pulse_len=n_chans}
      mask prompts: pulse_len "Length of Pulse"
      mask help:
      | Extends a boolean signal to be high for the specified number of clocks after
      | the last high input.
      mask init:
      | bits = ceil(log2(pulse_len+1));
      mask Help: eval('xlWeb([getenv(''MLIB_ROOT''), ''\casper_library\doc\pulse_ext_usage.html''])')
  zero : xbsIndex_r4/Constant  arith_type=Signed (2's comp)  const=0  n_bits=32  bin_pt=6  explicit_period=on  period=1  equ=P=C  opselect=C  inp2=PCIN>>17  opr=+  inp1=P  carry=CIN  dbl_ovrd=off  block_type=constant
  dout : Outport  OutDataType=sfix(16)  OutScaling=2^0
  valid : Outport  Port=2  OutDataType=sfix(16)  OutScaling=2^0
  wires:
  Delay2/1 -> Adder0/2
  Delay1/1 -> Adder0/1
  Adder0/1 -> delay_bram/1(In1)
  delay_bram/1(Out1) -> dout/1, Mux0/2
  new_acc/1 -> pulse_ext/1(in)
  din/1 -> Delay1/1
  pulse_ext/1(out) -> valid/1, Mux0/1
  Mux0/1 -> Delay2/1
  zero/1 -> Mux0/3

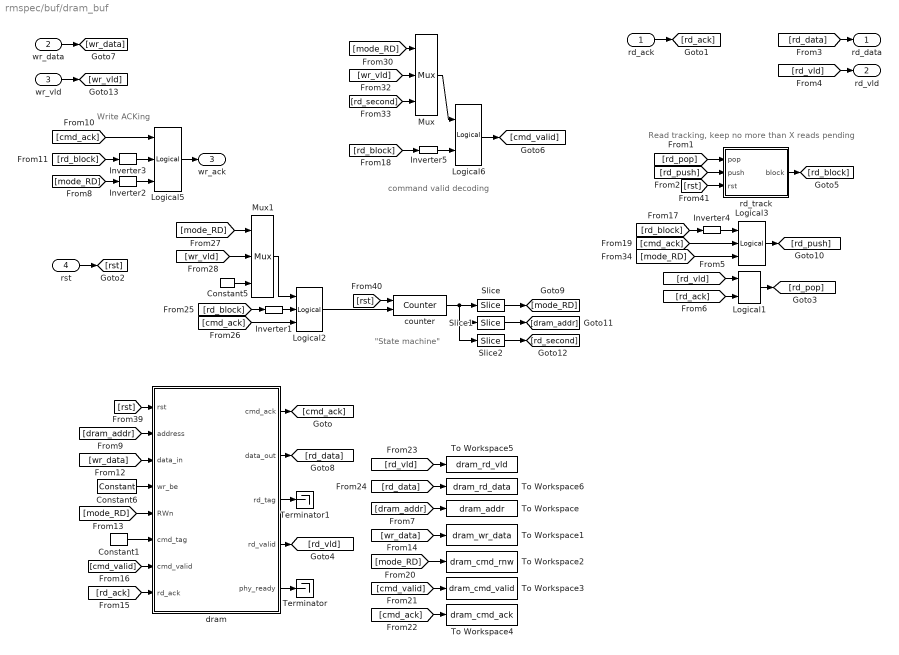
== system rmspec/buf/dram_buf ==
  note: Write ACKing
  note: "State machine"
  note: command valid decoding
  note: Read tracking, keep no more than X reads pending
  rd_ack : Inport  OutDataType=sfix(16)  OutScaling=2^0
  wr_data : Inport  Port=2  OutDataType=sfix(16)  OutScaling=2^0
  wr_vld : Inport  Port=3  OutDataType=sfix(16)  OutScaling=2^0
  rst : Inport  Port=4  OutDataType=sfix(16)  OutScaling=2^0
  Constant1 : xbsIndex_r4/Constant  arith_type=Unsigned  const=0  n_bits=32  bin_pt=0  explicit_period=on  period=1  equ=P=C  opselect=C  inp2=PCIN>>17  opr=+  inp1=P  carry=CIN  dbl_ovrd=off  block_type=constant
  Constant5 : xbsIndex_r4/Constant  arith_type=Boolean  const=1  n_bits=32  bin_pt=0  explicit_period=on  period=1  equ=P=C  opselect=C  inp2=PCIN>>17  opr=+  inp1=P  carry=CIN  dbl_ovrd=off  block_type=constant
  Constant6 : xbsIndex_r4/Constant  arith_type=Unsigned  const=2^18 - 1  n_bits=18  bin_pt=0  explicit_period=on  period=1  equ=P=C  opselect=C  inp2=PCIN>>17  opr=+  inp1=P  carry=CIN  dbl_ovrd=off  block_type=constant
  Inverter{1..5} (5 alike) : xbsIndex_r4/Inverter  en=off  latency=0  dbl_ovrd=off  block_type=inv
  Logical1 : xbsIndex_r4/Logical  logical_function=AND  inputs=2  en=off  latency=0  precision=Full  arith_type=Unsigned  n_bits=16  bin_pt=0  align_bp=on  dbl_ovrd=off  block_type=logical
  Logical2 : xbsIndex_r4/Logical  logical_function=AND  inputs=3  en=off  latency=0  precision=Full  arith_type=Unsigned  n_bits=16  bin_pt=0  align_bp=on  dbl_ovrd=off  block_type=logical
  Logical3 : xbsIndex_r4/Logical  logical_function=AND  inputs=3  en=off  latency=0  precision=Full  arith_type=Unsigned  n_bits=16  bin_pt=0  align_bp=on  dbl_ovrd=off  block_type=logical
  Logical5 : xbsIndex_r4/Logical  logical_function=AND  inputs=3  en=off  latency=0  precision=Full  arith_type=Unsigned  n_bits=16  bin_pt=0  align_bp=on  dbl_ovrd=off  block_type=logical
  Logical6 : xbsIndex_r4/Logical  logical_function=AND  inputs=2  en=off  latency=0  precision=Full  arith_type=Unsigned  n_bits=16  bin_pt=0  align_bp=on  dbl_ovrd=off  block_type=logical
  Mux : xbsIndex_r4/Mux  inputs=2  en=off  latency=0  precision=Full  arith_type=Unsigned  n_bits=16  bin_pt=14  quantization=Truncate  overflow=Wrap  dbl_ovrd=off  block_type=mux
  Mux1 : xbsIndex_r4/Mux  inputs=2  en=off  latency=0  precision=Full  arith_type=Unsigned  n_bits=16  bin_pt=14  quantization=Truncate  overflow=Wrap  dbl_ovrd=off  block_type=mux
  Slice : xbsIndex_r4/Slice  nbits=1  boolean_output=on  mode=Upper Bit Location + Width  bit1=0  base1=MSB of Input  bit0=0  base0=LSB of Input  dbl_ovrd=off  block_type=slice
      settings: infoedit="Extracts a given range of bits from each input sample and presents it at the output.  The output type is ordinarily unsigned with binary point at zero, but can be Boolean when the slice is one bit wide.<P><P>Hardware notes: In hardware this block costs nothing."  block_version=10.1.3
  Slice1 : xbsIndex_r4/Slice  nbits=block_size - 1  boolean_output=off  mode=Lower Bit Location + Width  bit1=0  base1=LSB of Input  bit0=1  base0=LSB of Input  dbl_ovrd=off  block_type=slice
      settings: infoedit="Extracts a given range of bits from each input sample and presents it at the output.  The output type is ordinarily unsigned with binary point at zero, but can be Boolean when the slice is one bit wide.<P><P>Hardware notes: In hardware this block costs nothing."  block_version=10.1.3
  Slice2 : xbsIndex_r4/Slice  nbits=1  boolean_output=on  mode=Lower Bit Location + Width  bit1=0  base1=LSB of Input  bit0=0  base0=LSB of Input  dbl_ovrd=off  block_type=slice
      settings: infoedit="Extracts a given range of bits from each input sample and presents it at the output.  The output type is ordinarily unsigned with binary point at zero, but can be Boolean when the slice is one bit wide.<P><P>Hardware notes: In hardware this block costs nothing."  block_version=10.1.3
  Terminator : Terminator
  Terminator1 : Terminator
  To Workspace : ToWorkspace  VariableName=dram_addr  SampleTime=-1  SaveFormat=Array
  To Workspace1 : ToWorkspace  VariableName=dram_wr_data  SampleTime=-1  SaveFormat=Array
  To Workspace2 : ToWorkspace  VariableName=dram_cmd_rnw  SampleTime=-1  SaveFormat=Array
  To Workspace3 : ToWorkspace  VariableName=dram_cmd_valid  SampleTime=-1  SaveFormat=Array
  To Workspace4 : ToWorkspace  VariableName=dram_cmd_ack  SampleTime=-1  SaveFormat=Array
  To Workspace5 : ToWorkspace  VariableName=dram_rd_vld  SampleTime=-1  SaveFormat=Array
  To Workspace6 : ToWorkspace  VariableName=dram_rd_data  SampleTime=-1  SaveFormat=Array
  counter : xbsIndex_r4/Counter  cnt_type=Free Running  cnt_to=Inf  operation=Up  start_count=0  cnt_by_val=1  arith_type=Unsigned  n_bits=block_size+1  bin_pt=0  load_pin=off  rst=on  en=on  explicit_period=on  period=1  dbl_ovrd=off  use_behavioral_HDL=off  use_rpm=off  implementation=Fabric  block_type=counter
  dram : Subsystem  Tag=xps:dram  AncestorBlock=xps_library/dram  mask(dram){dimm=1, arith_type=Unsigned, bin_pt=0, ip_clock=266, sample_period=1, bram_fifos=off, disable_tag=off, use_sim=off, ram_depth=18, bank_mgt=off, wide_data=off, half_burst=off, use_sniffer=off}
      mask prompts: arith_type "Data Type"; bin_pt "Data binary point"; ip_clock "Datapath clock rate (MHz)"; sample_period "Sample period"; bram_fifos "Use BRAM FIFOs"; disable_tag "Disable tag FIFO"; use_sim "Simulate DRAM using ModelSim"; ram_depth "Lesser simulation address width"; bank_mgt "Enable bank management"; wide_data "Use wide data bus (288 bits)"; half_burst "Use half-burst"; use_sniffer "Include CPU Interface"
      mask help:
      | Interface to 1GB DDR2 DIMMs on BEE2.
      |
      | To simulate using ModelSim, place a ModelSim block named 'ModelSim' (case-sensitive) in the top level of the design.
      |
      | Commands that are clocked-in are executed with an unknown delay, however, execution order is maintained.
      mask init:
      | dram_mask(gcb, use_sim, wide_data);
      mask Help: eval('xlWeb([getenv(''MLIB_ROOT''), ''\doc\html\sys_dram\sys_dram.html''])')
      mask StyleString: popup(1|2|3|4),popup(Boolean|Unsigned|Signed  (2's comp)),edit,edit,edit,checkbox,checkbox,checkbox,edit,checkbox,checkbox,checkbox,checkbox
      mask CallbackString:
      | |||||||myname=gcb;
      | if strcmp(get_param(myname, 'use_sim'), 'off')
      |     masks = get_param(myname, 'MaskEnables');
      |     masks{9} = 'on';
      |     set_param(myname, 'MaskEnables', masks);
      | else
      |     masks = get_param(myname, 'MaskEnables');
      |     masks{9} = 'off';
      |     set_param(myname, 'MaskEnables', masks);
      | end|||myname=gcb;
      | if strcmp(get_param(myname, 'wide_data'), 'off')
      |     masks = get_param(myname, 'MaskEnables');
      |     masks{12} = 'on';
      |     set_param(myname, 'MaskEnables', masks);
      | else
      |     set_param(myname, 'half_burst', 'off');
      |     masks = get_param(myname, 'MaskEnables');
      |     masks{12} = 'off';
      |     set_param(myname, 'MaskEnables', masks);
      | end||
  rd_track : Subsystem  mask{max=16}
  rd_data : Outport  OutDataType=sfix(16)  OutScaling=2^0
  rd_vld : Outport  Port=2  OutDataType=sfix(16)  OutScaling=2^0
  wr_ack : Outport  Port=3  OutDataType=sfix(16)  OutScaling=2^0
  wires:
  [rd_data] -> To Workspace6/1
  [rd_vld] -> To Workspace5/1
  [cmd_ack] -> To Workspace4/1
  [cmd_valid] -> To Workspace3/1
  [mode_RD] -> To Workspace2/1
  [wr_data] -> To Workspace1/1
  [wr_data] -> dram/3(data_in)
  wr_data/1 -> [wr_data]
  [dram_addr] -> To Workspace/1
  Logical6/1 -> [cmd_valid]
  Inverter5/1 -> Logical6/2
  [rd_block] -> Inverter5/1
  [cmd_valid] -> dram/7(cmd_valid)
  Constant1/1 -> dram/6(cmd_tag)
  [mode_RD] -> dram/5(RWn)
  [rd_ack] -> dram/8(rd_ack)
  Logical5/1 -> wr_ack/1
  [mode_RD] -> Inverter2/1
  Inverter3/1 -> Logical5/2
  [rd_block] -> Inverter3/1
  [cmd_ack] -> Logical5/1
  dram/4(rd_valid) -> [rd_vld]
  dram/2(data_out) -> [rd_data]
  dram/3(rd_tag) -> Terminator1/1
  dram/5(phy_ready) -> Terminator/1
  dram/1(cmd_ack) -> [cmd_ack]
  [dram_addr] -> dram/2(address)
  rd_ack/1 -> [rd_ack]
  rd_track/1(block) -> [rd_block]
  [rst] -> dram/1(rst)
  Constant6/1 -> dram/4(wr_be)
  [rd_pop] -> rd_track/1(pop)
  [rd_push] -> rd_track/2(push)
  [rd_data] -> rd_data/1
  [rd_vld] -> rd_vld/1
  [rd_vld] -> Logical1/1
  [rd_ack] -> Logical1/2
  Logical1/1 -> [rd_pop]
  counter/1 -> Slice/1, Slice1/1, Slice2/1
  Slice/1 -> [mode_RD]
  Slice1/1 -> [dram_addr]
  Inverter2/1 -> Logical5/3
  Slice2/1 -> [rd_second]
  Mux/1 -> Logical6/1
  [mode_RD] -> Mux/1
  wr_vld/1 -> [wr_vld]
  [wr_vld] -> Mux/2
  [rd_second] -> Mux/3
  [rd_block] -> Inverter4/1
  Inverter4/1 -> Logical3/1
  [cmd_ack] -> Logical3/2
  [mode_RD] -> Logical3/3
  Logical3/1 -> [rd_push]
  [rd_block] -> Inverter1/1
  Inverter1/1 -> Logical2/2
  [cmd_ack] -> Logical2/3
  Mux1/1 -> Logical2/1
  [mode_RD] -> Mux1/1
  [wr_vld] -> Mux1/2
  Constant5/1 -> Mux1/3
  Logical2/1 -> counter/2
  rst/1 -> [rst]
  [rst] -> rd_track/3(rst)
  [rst] -> counter/1
